simulink library "ddm"  (R2021b)
settings: Solver=VariableStepAuto  StartTime=0.0  StopTime=10.0  RelTol=1e-3
undefined symbols (not defined in the file or in its folder): ENUM_ADASACCSTA_ERROR, ENUM_ADASACCSTA_OFF, ENUM_ADASACCSTA_STANDBY, ENUM_ADASISASTA_OFF, ENUM_ALLOWMOV_ALLOWREADY, ENUM_APS, ENUM_BRKSTA_ERROR, ENUM_BRKSTA_OFF, ENUM_BRKSTA_ON, ENUM_CHGPREACTERRSTA_OBCPRE, ENUM_DCDCFAULTSTA_ANYFAULTLV1, ENUM_DCDCFAULTSTA_ANYFAULTLV2, ENUM_DRIVETRAIN_AWD, ENUM_DRIVETRAIN_FWD, ENUM_DRIVETRAIN_RWD, ENUM_DRSEATSTA_INVALID, ENUM_EDUDRTSTA_NORMAL, ENUM_EPBSTA_APPLIED, ENUM_EPBSTA_RELEASED, ENUM_HVBATTREADYPRE_READY, ENUM_MCUWARN_LV0, ENUM_MCUWARN_LV1, ENUM_MCUWARN_LV2, ENUM_MCUWARN_LV3, ENUM_MCUWARN_NOERROR, ENUM_OBCFAULTSTA_ANYFAULT, ENUM_PAS_R2F2, ENUM_PDFAULT_BATTPDFAIL, ENUM_PDFAULT_DCDCDISABLE, ENUM_PDFAULT_MCUDISABLE, ENUM_PDFAULT_MCUDISCHRG, ENUM_POWERSTA_OFF, ENUM_POWERSTA_ON, ENUM_POWERSTA_READY, ENUM_POWERSTA_STANDBY, ENUM_PRESSINDI_LOW, ENUM_PUFAULT_BATTUPFAIL, ENUM_PUFAULT_DCDCENABLEFAIL, ENUM_PUFAULT_PRECHRGCHKFAIL, ENUM_PUFAULT_SAFETYCHKFAIL, ENUM_PUSTATE_COMPLETED, ENUM_PWRSTASW_OFF, ENUM_PWRSTASW_OFFA, ENUM_PWRSTASW_OFFCHVCHRG, ENUM_PWRSTASW_OFFCLVCHRG, ENUM_PWRSTASW_ON, ENUM_PWRSTASW_ONHVCHRG, ENUM_PWRSTASW_READY, ENUM_PWRSTASW_STANDBY, ENUM_RANGESTA_12IN, ENUM_RANGESTA_12OUT, ENUM_SHIFTCOMMAND_D, ENUM_SHIFTCOMMAND_N, ENUM_SHIFTCOMMAND_P, ENUM_SHIFTCOMMAND_R, ENUM_ZONEMALFUNLV_1ST, ENUM_ZONEMALFUNLV_2ND, ENUM_ZONEMALFUNLV_3RD, ENUM_ZONEMALFUNLV_4TH, ENUM_ZONESPDCTRLMODE_ACC ... (+832)
libraries: hcu_lib x738, $bdroot x26, simulink x7
(part 13 of 25)

== system ddm/DDM/DDM/PMM/Comm err/FDC lost communication with EPAS2 ==
  note: Fail Safe After Decision
  note: Test Pass Criteria
  note: Diagnostics and Fault Handling
  note: Test Detection Criteria
  note: Fail Safe During Detection
  note: Release Condition After Failure Decision
  note: Release Condition During Failure Detection
  task_time_s : Inport
  VPMM_PowerSta_enum : Inport  Port=2
  VPMM_PwrStaSW_enum : Inport  Port=3
  VDDM_C1EPAS2LCChk_flg : Inport  Port=4
  No_CAN1_BUS_OFF : Inport  Port=5
  DTC_clear_request : Inport  Port=6
  Constant15 : Constant  Value=KDDM_C1EPAS2LCCFSSW_flg
  Constant16 : Constant  Value=TRUE
  Constant18 : Constant  Value=KDDM_C1EPAS2LCPassTO_s
  Constant19 : Constant  Value=KDDM_C1EPAS2LCPassTO_s
  Constant{2,21,25,27} (4 alike) : Constant  Value=FALSE
  Constant20 : Constant  Value=KDDM_C1EPAS2LCDFSSW_flg
  Constant24 : Constant  Value=TRUE
  Constant26 : Constant  Value=ENUM_PWRSTASW_OFF
  Constant28 : Constant  Value=ENUM_PWRSTASW_OFF
  Constant3 : Constant  Value=TRUE
  Constant4 : Constant  Value=ENUM_POWERSTA_OFF
  Constant40 : Constant  Value=KDDM_C1EPAS2LCDTC_cnt
  Constant41 : Constant  Value=KDDM_C1EPAS2LCDetTO_s
  Constant46 : Constant  Value=KDDM_C1EPAS2LCDetSW_flg
  Constant48 : Constant  Value=KDDM_C1EPAS2LCDTC_cnt
  Constant5 : Constant  Value=KDDM_C1EPAS2LCPassSW_flg
  DTC_Couter : hcu_lib/Basic_Blocks/DTC_Couter
  DTC_Info : hcu_lib/Basic_Blocks/DTC_Info
  Data Type Conversion1 : DataTypeConversion  OutDataTypeStr=uint8
  Equal : RelationalOperator  Operator=~=  OutDataTypeStr=boolean  RndMeth=Simplest
  Equal2 : RelationalOperator  Operator=~=  OutDataTypeStr=boolean  RndMeth=Simplest
  Equal3 : RelationalOperator  OutDataTypeStr=boolean  RndMeth=Simplest
  Equal4 : RelationalOperator  Operator===  OutDataTypeStr=boolean  RndMeth=Simplest
  Goto19 : Goto  Commented=on  GotoTag=EDriveSysErr_VCUErr_flg
  Logical Operator{2,5,12,15,18..19} (6 alike) : Logic  AllPortsSameDT=off  OutDataTypeStr=boolean
  Logical Operator3 : Logic  Operator=OR  AllPortsSameDT=off  OutDataTypeStr=boolean
  Logical Operator6 : Logic  Operator=NOT  AllPortsSameDT=off  OutDataTypeStr=boolean
  Logical Operator8 : Logic  Operator=OR  AllPortsSameDT=off  OutDataTypeStr=boolean
  Relay : Relay  OnSwitchValue=ONE_INT  OffSwitchValue=ZERO_INT
  SR_Latch1 : Subsystem  mask(SR_Latch){}
      mask help: SR latch function.
  SR_Latch3 : hcu_lib/Basic_Blocks/SR_Latch
  SR_Latch4 : hcu_lib/Basic_Blocks/SR_Latch
  Switch{,1,4..6} (5 alike) : Switch  Criteria=u2 ~= 0
  Test Detection Criteria : hcu_lib/Basic_Blocks/Test Detection Criteria
  Timer1 : hcu_lib/Basic_Blocks/Timer
  VDDM_C1EPAS2LCDTC_raw32 : Outport
  VDDM_C1EPAS2LCCFS_flg : Outport  Port=2
  wires:
  Constant2/1 -> Switch1/1
  Switch5/1 -> Switch1/3, [VDDM_xxx_flg]
  Switch1/1 -> Test Detection Criteria/1
  [DTC_clear_request] -> Switch1/2
  [DTC_clear_request] -> DTC_Info/4
  Constant41/1 -> Test Detection Criteria/4
  [VDDM_C1EPAS2LCPass_flg] -> DTC_Info/2
  [VDDM_C1EPAS2LCDet_flg] -> DTC_Info/1
  [VDDM_C1EPAS2LCCFS_flg] -> SR_Latch3/2
  [VDDM_C1EPAS2LCCFS_flg] -> VDDM_C1EPAS2LCCFS_flg/1, DTC_Info/3
  DTC_Info/1 -> VDDM_C1EPAS2LCDTC_raw32/1  "VDDM_C1EPAS2LCDTC_raw32"
  [task_time_s] -> Timer1/3
  [VPMM_PwrStaSW_enum] -> Equal2/1
  [VPMM_PwrStaSW_enum] -> Equal/1
  [VPMM_PowerSta_enum] -> Equal4/1
  Constant4/1 -> Equal4/2
  [VDDM_C1EPAS2LCPass_flg] -> Logical Operator3/1
  Constant18/1 -> Timer1/4
  [VDDM_C1EPAS2LCDet_flg] -> Logical Operator19/1
  Equal3/1 -> SR_Latch1/1(set)
  Logical Operator18/1 -> [VDDM_C1EPAS2LCCFS_flg]
  Switch6/1 -> Timer1/2, Logical Operator6/1
  SR_Latch1/1(latched) -> [VDDM_C1EPAS2LCPass_flg]
  Constant48/1 -> DTC_Couter/3
  SR_Latch4/1 -> Logical Operator18/1
  Constant28/1 -> Equal2/2
  DTC_Couter/2 -> Data Type Conversion1/1
  [VDDM_C1EPAS2LCChk_flg] -> Switch5/1
  Logical Operator15/1 -> DTC_Couter/2
  Logical Operator3/1 -> Logical Operator15/1
  Logical Operator8/1 -> Switch4/2
  Constant15/1 -> Logical Operator18/2
  [VDDM_C1EPAS2LCChk_flg] -> Switch6/1
  Switch4/1 -> [VDDM_C1EPAS2LCCFSRls_flg]
  Logical Operator19/1 -> DTC_Couter/1
  Constant25/1 -> Switch4/3
  Equal2/1 -> Logical Operator5/2
  Constant20/1 -> Logical Operator12/1
  [VDDM_C1EPAS2LCCFS_flg] -> Switch/2
  Constant21/1 -> Switch/3
  DTC_Couter/1 -> SR_Latch4/1
  Logical Operator12/1 -> [VDDM_C1EPAS2LCDFS_flg]
  Constant40/1 -> Test Detection Criteria/3
  [VDDM_xxx_flg] -> SR_Latch1/2(reset)
  [No_CAN1_BUS_OFF] -> Logical Operator5/1
  [VDDM_C1EPAS2LCCFSRls_flg] -> Logical Operator3/2
  Relay/1 -> SR_Latch3/1
  Switch/1 -> Goto19/1
  Logical Operator5/1 -> Switch6/2
  Logical Operator2/1 -> Switch5/2
  Constant24/1 -> Switch4/1
  Constant46/1 -> Logical Operator19/2
  SR_Latch3/1 -> Logical Operator12/2
  Constant5/1 -> Logical Operator15/2
  [VDDM_C1EPAS2LCCFSRls_flg] -> SR_Latch4/2
  Constant26/1 -> Equal/2
  [DTC_clear_request] -> Logical Operator8/2
  Data Type Conversion1/1 -> [VDDM_C1EPAS2LCDTC_cnt]  "VDDM_C1EPAS2LCDTC_cnt"
  [No_CAN1_BUS_OFF] -> Logical Operator2/1
  Constant27/1 -> Switch5/3
  Timer1/1 -> Equal3/1
  Equal4/1 -> Logical Operator8/1
  Equal/1 -> Logical Operator2/2
  [task_time_s] -> Test Detection Criteria/2
  Logical Operator6/1 -> Timer1/1
  [VDDM_C1EPAS2LCDTC_cnt] -> Relay/1
  Constant16/1 -> Switch6/3
  Constant19/1 -> Equal3/2
  Constant3/1 -> Switch/1
  No_CAN1_BUS_OFF/1 -> [No_CAN1_BUS_OFF]
  DTC_clear_request/1 -> [DTC_clear_request]
  task_time_s/1 -> [task_time_s]
  VDDM_C1EPAS2LCChk_flg/1 -> [VDDM_C1EPAS2LCChk_flg]
  VPMM_PwrStaSW_enum/1 -> [VPMM_PwrStaSW_enum]
  VPMM_PowerSta_enum/1 -> [VPMM_PowerSta_enum]
  Test Detection Criteria/1 -> [VDDM_C1EPAS2LCDet_flg]  "VDDM_C1EPAS2LCDet_flg"

== system ddm/DDM/DDM/PMM/Comm err/The CAN signal between VCU and ABM1 is discontinuous ==
  note: Fail Safe During Detection
  note: Diagnostics and Fault Handling
  note: Test Pass Criteria
  note: Test Detection Criteria
  note: Release Condition During Failure Detection
  note: Fail Safe After Decision
  note: Release Condition After Failure Decision
  task_time_s : Inport
  VPMM_PowerSta_enum : Inport  Port=2
  VPMM_PwrStaSW_enum : Inport  Port=3
  VDDM_C1ABM1RCChk_flg : Inport  Port=4
  VDDM_C1ABM1LCCFS_flg : Inport  Port=5
  No_CAN1_BUS_OFF : Inport  Port=6
  DTC_clear_request : Inport  Port=7
  Constant15 : Constant  Value=KDDM_C1ABM1RCCFSSW_flg
  Constant16 : Constant  Value=TRUE
  Constant18 : Constant  Value=KDDM_C1ABM1RCPassTO_s
  Constant19 : Constant  Value=KDDM_C1ABM1RCPassTO_s
  Constant{2,21,25,27} (4 alike) : Constant  Value=FALSE
  Constant20 : Constant  Value=KDDM_C1ABM1RCDFSSW_flg
  Constant24 : Constant  Value=TRUE
  Constant26 : Constant  Value=ENUM_PWRSTASW_OFF
  Constant28 : Constant  Value=ENUM_PWRSTASW_OFF
  Constant3 : Constant  Value=TRUE
  Constant4 : Constant  Value=ENUM_POWERSTA_OFF
  Constant40 : Constant  Value=KDDM_C1ABM1RCDTC_cnt
  Constant41 : Constant  Value=KDDM_C1ABM1RCDetTO_s
  Constant46 : Constant  Value=KDDM_C1ABM1RCDetSW_flg
  Constant48 : Constant  Value=KDDM_C1ABM1RCDTC_cnt
  Constant5 : Constant  Value=KDDM_C1ABM1RCPassSW_flg
  DTC_Couter : hcu_lib/Basic_Blocks/DTC_Couter
  DTC_Info : hcu_lib/Basic_Blocks/DTC_Info
  Data Type Conversion1 : DataTypeConversion  OutDataTypeStr=uint8
  Equal : RelationalOperator  Operator=~=  OutDataTypeStr=boolean  RndMeth=Simplest
  Equal2 : RelationalOperator  Operator=~=  OutDataTypeStr=boolean  RndMeth=Simplest
  Equal3 : RelationalOperator  OutDataTypeStr=boolean  RndMeth=Simplest
  Equal4 : RelationalOperator  Operator===  OutDataTypeStr=boolean  RndMeth=Simplest
  Logical Operator1 : Logic  Operator=NOT  AllPortsSameDT=off  OutDataTypeStr=boolean
  Logical Operator{12,15,18..19} (4 alike) : Logic  AllPortsSameDT=off  OutDataTypeStr=boolean
  Logical Operator2 : Logic  Inputs=3  AllPortsSameDT=off  OutDataTypeStr=boolean
  Logical Operator3 : Logic  Operator=OR  AllPortsSameDT=off  OutDataTypeStr=boolean
  Logical Operator4 : Logic  Operator=NOT  AllPortsSameDT=off  OutDataTypeStr=boolean
  Logical Operator5 : Logic  Inputs=3  AllPortsSameDT=off  OutDataTypeStr=boolean
  Logical Operator6 : Logic  Operator=NOT  AllPortsSameDT=off  OutDataTypeStr=boolean
  Logical Operator8 : Logic  Operator=OR  AllPortsSameDT=off  OutDataTypeStr=boolean
  Relay : Relay  OnSwitchValue=ONE_INT  OffSwitchValue=ZERO_INT
  SR_Latch1 : Subsystem  mask(SR_Latch){}
      mask help: SR latch function.
  SR_Latch3 : hcu_lib/Basic_Blocks/SR_Latch
  SR_Latch4 : hcu_lib/Basic_Blocks/SR_Latch
  Switch{,1,4..6} (5 alike) : Switch  Criteria=u2 ~= 0
  Test Detection Criteria : hcu_lib/Basic_Blocks/Test Detection Criteria
  Timer1 : hcu_lib/Basic_Blocks/Timer
  VDDM_C1ABM1RCDTC_raw32 : Outport
  RC_EDriveSysErr_VCUErr_flg : Outport  Port=2
  wires:
  task_time_s/1 -> [task_time_s]
  VDDM_C1ABM1RCChk_flg/1 -> [VDDM_C1ABM1RCChk_flg]
  VPMM_PwrStaSW_enum/1 -> [VPMM_PwrStaSW_enum]
  VPMM_PowerSta_enum/1 -> [VPMM_PowerSta_enum]
  VDDM_C1ABM1LCCFS_flg/1 -> [VDDM_C1ABM1LCCFS_flg]
  No_CAN1_BUS_OFF/1 -> [No_CAN1_BUS_OFF]
  DTC_clear_request/1 -> [DTC_clear_request]
  Equal2/1 -> Logical Operator5/2
  SR_Latch1/1(latched) -> [VDDM_C1ABM1RCPass_flg]
  SR_Latch4/1 -> Logical Operator18/1
  Constant20/1 -> Logical Operator12/1
  Logical Operator19/1 -> DTC_Couter/1
  Constant48/1 -> DTC_Couter/3
  [No_CAN1_BUS_OFF] -> Logical Operator5/1
  Data Type Conversion1/1 -> [VDDM_C1ABM1RCDTC_cnt]  "VDDM_C1ABM1RCDTC_cnt"
  Constant27/1 -> Switch5/3
  Switch6/1 -> Logical Operator6/1, Timer1/2
  Switch4/1 -> [VDDM_C1ABM1RCCFSRls_flg]
  Constant24/1 -> Switch4/1
  [VDDM_C1ABM1RCCFS_flg] -> Switch/2
  Constant5/1 -> Logical Operator15/2
  Constant3/1 -> Switch/1
  Constant18/1 -> Timer1/4
  [VDDM_C1ABM1LCCFS_flg] -> Logical Operator1/1
  Test Detection Criteria/1 -> [VDDM_C1ABM1RCDet_flg]  "VDDM_C1ABM1RCDet_flg"
  Constant46/1 -> Logical Operator19/2
  SR_Latch3/1 -> Logical Operator12/2
  Logical Operator4/1 -> Logical Operator5/3
  [VDDM_C1ABM1RCChk_flg] -> Switch5/1
  Constant40/1 -> Test Detection Criteria/3
  Constant26/1 -> Equal/2
  Logical Operator3/1 -> Logical Operator15/1
  [VDDM_C1ABM1RCDTC_cnt] -> Relay/1
  Constant19/1 -> Equal3/2
  Equal4/1 -> Logical Operator8/1
  [No_CAN1_BUS_OFF] -> Logical Operator2/1
  Constant25/1 -> Switch4/3
  Logical Operator2/1 -> Switch5/2
  Constant16/1 -> Switch6/3
  Logical Operator12/1 -> [VDDM_C1ABM1RCDFS_flg]
  [DTC_clear_request] -> Logical Operator8/2
  Relay/1 -> SR_Latch3/1
  Constant21/1 -> Switch/3
  Switch/1 -> [EDriveSysErr_VCUErr_flg]
  [VDDM_C1ABM1RCCFSRls_flg] -> Logical Operator3/2
  [VDDM_xxx_flg] -> SR_Latch1/2(reset)
  [VDDM_C1ABM1LCCFS_flg] -> Logical Operator4/1
  [task_time_s] -> Test Detection Criteria/2
  Logical Operator1/1 -> Logical Operator2/3
  Equal3/1 -> SR_Latch1/1(set)
  Timer1/1 -> Equal3/1
  [VDDM_C1ABM1RCChk_flg] -> Switch6/1
  Constant15/1 -> Logical Operator18/2
  Logical Operator6/1 -> Timer1/1
  Logical Operator5/1 -> Switch6/2
  Constant28/1 -> Equal2/2
  DTC_Couter/1 -> SR_Latch4/1
  Equal/1 -> Logical Operator2/2
  Logical Operator15/1 -> DTC_Couter/2
  [VDDM_C1ABM1RCDet_flg] -> Logical Operator19/1
  Logical Operator18/1 -> [VDDM_C1ABM1RCCFS_flg]
  Logical Operator8/1 -> Switch4/2
  Constant4/1 -> Equal4/2
  [VDDM_C1ABM1RCCFSRls_flg] -> SR_Latch4/2
  DTC_Couter/2 -> Data Type Conversion1/1
  [VDDM_C1ABM1RCPass_flg] -> Logical Operator3/1
  [EDriveSysErr_VCUErr_flg] -> RC_EDriveSysErr_VCUErr_flg/1
  [VPMM_PowerSta_enum] -> Equal4/1
  [VPMM_PwrStaSW_enum] -> Equal/1
  [VPMM_PwrStaSW_enum] -> Equal2/1
  [task_time_s] -> Timer1/3
  DTC_Info/1 -> VDDM_C1ABM1RCDTC_raw32/1  "VDDM_C1ABM1RCDTC_raw32"
  [VDDM_C1ABM1RCPass_flg] -> DTC_Info/2
  [VDDM_C1ABM1RCCFS_flg] -> DTC_Info/3
  [VDDM_C1ABM1RCCFS_flg] -> SR_Latch3/2
  [VDDM_C1ABM1RCDet_flg] -> DTC_Info/1
  Constant41/1 -> Test Detection Criteria/4
  [DTC_clear_request] -> DTC_Info/4
  [DTC_clear_request] -> Switch1/2
  Switch1/1 -> Test Detection Criteria/1
  Switch5/1 -> [VDDM_xxx_flg], Switch1/3
  Constant2/1 -> Switch1/1

== system ddm/DDM/DDM/PMM/Comm err/The CAN signal between VCU and ABM1 is incomplete ==
  note: Diagnostics and Fault Handling
  note: Fail Safe During Detection
  note: Release Condition After Failure Decision
  note: Fail Safe After Decision
  note: Release Condition During Failure Detection
  note: Test Detection Criteria
  note: Test Pass Criteria
  task_time_s : Inport
  VPMM_PowerSta_enum : Inport  Port=2
  VPMM_PwrStaSW_enum : Inport  Port=3
  VDDM_C1ABM1CSChk_flg : Inport  Port=4
  VDDM_C1ABM1LCCFS_flg : Inport  Port=5
  No_CAN1_BUS_OFF : Inport  Port=6
  DTC_clear_request : Inport  Port=7
  Constant15 : Constant  Value=KDDM_C1ABM1CSCFSSW_flg
  Constant16 : Constant  Value=TRUE
  Constant18 : Constant  Value=KDDM_C1ABM1CSPassTO_s
  Constant19 : Constant  Value=KDDM_C1ABM1CSPassTO_s
  Constant{2,21,25,27} (4 alike) : Constant  Value=FALSE
  Constant20 : Constant  Value=KDDM_C1ABM1CSDFSSW_flg
  Constant24 : Constant  Value=TRUE
  Constant26 : Constant  Value=ENUM_PWRSTASW_OFF
  Constant28 : Constant  Value=ENUM_PWRSTASW_OFF
  Constant3 : Constant  Value=TRUE
  Constant4 : Constant  Value=ENUM_POWERSTA_OFF
  Constant40 : Constant  Value=KDDM_C1ABM1CSDTC_cnt
  Constant41 : Constant  Value=KDDM_C1ABM1CSDetTO_s
  Constant46 : Constant  Value=KDDM_C1ABM1CSDetSW_flg
  Constant48 : Constant  Value=KDDM_C1ABM1CSDTC_cnt
  Constant5 : Constant  Value=KDDM_C1ABM1CSPassSW_flg
  DTC_Couter : hcu_lib/Basic_Blocks/DTC_Couter
  DTC_Info : hcu_lib/Basic_Blocks/DTC_Info
  Data Type Conversion1 : DataTypeConversion  OutDataTypeStr=uint8
  Equal : RelationalOperator  Operator=~=  OutDataTypeStr=boolean  RndMeth=Simplest
  Equal2 : RelationalOperator  Operator=~=  OutDataTypeStr=boolean  RndMeth=Simplest
  Equal3 : RelationalOperator  OutDataTypeStr=boolean  RndMeth=Simplest
  Equal4 : RelationalOperator  Operator===  OutDataTypeStr=boolean  RndMeth=Simplest
  Logical Operator1 : Logic  Operator=NOT  AllPortsSameDT=off  OutDataTypeStr=boolean
  Logical Operator{12,15,18..19} (4 alike) : Logic  AllPortsSameDT=off  OutDataTypeStr=boolean
  Logical Operator2 : Logic  Inputs=3  AllPortsSameDT=off  OutDataTypeStr=boolean
  Logical Operator3 : Logic  Operator=OR  AllPortsSameDT=off  OutDataTypeStr=boolean
  Logical Operator4 : Logic  Operator=NOT  AllPortsSameDT=off  OutDataTypeStr=boolean
  Logical Operator5 : Logic  Inputs=3  AllPortsSameDT=off  OutDataTypeStr=boolean
  Logical Operator6 : Logic  Operator=NOT  AllPortsSameDT=off  OutDataTypeStr=boolean
  Logical Operator8 : Logic  Operator=OR  AllPortsSameDT=off  OutDataTypeStr=boolean
  Relay : Relay  OnSwitchValue=ONE_INT  OffSwitchValue=ZERO_INT
  SR_Latch1 : Subsystem  mask(SR_Latch){}
      mask help: SR latch function.
  SR_Latch3 : hcu_lib/Basic_Blocks/SR_Latch
  SR_Latch4 : hcu_lib/Basic_Blocks/SR_Latch
  Switch{,1,4..6} (5 alike) : Switch  Criteria=u2 ~= 0
  Test Detection Criteria : hcu_lib/Basic_Blocks/Test Detection Criteria
  Timer1 : hcu_lib/Basic_Blocks/Timer
  VDDM_C1ABM1CSDTC_raw32 : Outport
  CS_EDriveSysErr_VCUErr_flg : Outport  Port=2
  wires:
  VDDM_C1ABM1LCCFS_flg/1 -> [VDDM_C1ABM1LCCFS_flg]
  VPMM_PowerSta_enum/1 -> [VPMM_PowerSta_enum]
  VPMM_PwrStaSW_enum/1 -> [VPMM_PwrStaSW_enum]
  VDDM_C1ABM1CSChk_flg/1 -> [VDDM_C1ABM1CSChk_flg]
  task_time_s/1 -> [task_time_s]
  DTC_clear_request/1 -> [DTC_clear_request]
  No_CAN1_BUS_OFF/1 -> [No_CAN1_BUS_OFF]
  SR_Latch4/1 -> Logical Operator18/1
  [VDDM_C1ABM1CSPass_flg] -> Logical Operator3/1
  DTC_Couter/2 -> Data Type Conversion1/1
  [VDDM_C1ABM1CSCFSRls_flg] -> SR_Latch4/2
  Constant4/1 -> Equal4/2
  [VDDM_C1ABM1CSDet_flg] -> Logical Operator19/1
  Logical Operator18/1 -> [VDDM_C1ABM1CSCFS_flg]
  Logical Operator15/1 -> DTC_Couter/2
  Equal2/1 -> Logical Operator5/2
  SR_Latch1/1(latched) -> [VDDM_C1ABM1CSPass_flg]
  Test Detection Criteria/1 -> [VDDM_C1ABM1CSDet_flg]  "VDDM_C1ABM1CSDet_flg"
  SR_Latch3/1 -> Logical Operator12/2
  [VDDM_C1ABM1LCCFS_flg] -> Logical Operator1/1
  Constant18/1 -> Timer1/4
  Logical Operator8/1 -> Switch4/2
  [VDDM_C1ABM1CSCFS_flg] -> Switch/2
  Constant5/1 -> Logical Operator15/2
  Constant24/1 -> Switch4/1
  Constant27/1 -> Switch5/3
  Switch4/1 -> [VDDM_C1ABM1CSCFSRls_flg]
  Switch6/1 -> Logical Operator6/1, Timer1/2
  Data Type Conversion1/1 -> [VDDM_C1ABM1CSDTC_cnt]  "VDDM_C1ABM1CSDTC_cnt"
  Constant20/1 -> Logical Operator12/1
  Logical Operator19/1 -> DTC_Couter/1
  DTC_Couter/1 -> SR_Latch4/1
  Constant28/1 -> Equal2/2
  Constant15/1 -> Logical Operator18/2
  [VDDM_C1ABM1CSChk_flg] -> Switch6/1
  Equal3/1 -> SR_Latch1/1(set)
  Constant48/1 -> DTC_Couter/3
  [task_time_s] -> Test Detection Criteria/2
  Logical Operator1/1 -> Logical Operator2/3
  Logical Operator5/1 -> Switch6/2
  [VDDM_C1ABM1LCCFS_flg] -> Logical Operator4/1
  [VDDM_xxx_flg] -> SR_Latch1/2(reset)
  [VDDM_C1ABM1CSCFSRls_flg] -> Logical Operator3/2
  Constant46/1 -> Logical Operator19/2
  Switch/1 -> [EDriveSysErr_VCUErr_flg]
  Constant21/1 -> Switch/3
  Logical Operator6/1 -> Timer1/1
  [DTC_clear_request] -> Logical Operator8/2
  Equal/1 -> Logical Operator2/2
  Logical Operator12/1 -> [VDDM_C1ABM1CSDFS_flg]
  Relay/1 -> SR_Latch3/1
  [No_CAN1_BUS_OFF] -> Logical Operator5/1
  Logical Operator2/1 -> Switch5/2
  Constant25/1 -> Switch4/3
  [No_CAN1_BUS_OFF] -> Logical Operator2/1
  Equal4/1 -> Logical Operator8/1
  Constant26/1 -> Equal/2
  Timer1/1 -> Equal3/1
  Logical Operator3/1 -> Logical Operator15/1
  Logical Operator4/1 -> Logical Operator5/3
  [VDDM_C1ABM1CSDTC_cnt] -> Relay/1
  [VDDM_C1ABM1CSChk_flg] -> Switch5/1
  Constant16/1 -> Switch6/3
  Constant40/1 -> Test Detection Criteria/3
  Constant19/1 -> Equal3/2
  Constant3/1 -> Switch/1
  [EDriveSysErr_VCUErr_flg] -> CS_EDriveSysErr_VCUErr_flg/1
  [VPMM_PowerSta_enum] -> Equal4/1
  [VPMM_PwrStaSW_enum] -> Equal/1
  [VPMM_PwrStaSW_enum] -> Equal2/1
  [task_time_s] -> Timer1/3
  DTC_Info/1 -> VDDM_C1ABM1CSDTC_raw32/1  "VDDM_C1ABM1CSDTC_raw32"
  [VDDM_C1ABM1CSCFS_flg] -> DTC_Info/3
  [VDDM_C1ABM1CSCFS_flg] -> SR_Latch3/2
  [VDDM_C1ABM1CSPass_flg] -> DTC_Info/2
  [VDDM_C1ABM1CSDet_flg] -> DTC_Info/1
  Constant41/1 -> Test Detection Criteria/4
  [DTC_clear_request] -> DTC_Info/4
  [DTC_clear_request] -> Switch1/2
  Switch1/1 -> Test Detection Criteria/1
  Switch5/1 -> [VDDM_xxx_flg], Switch1/3
  Constant2/1 -> Switch1/1

== system ddm/DDM/DDM/PMM/Comm err/The CAN signal between VCU and BMS1 is discontinuous ==
  note: Test Pass Criteria
  note: Release Condition After Failure Decision
  note: Diagnostics and Fault Handling
  note: Release Condition During Failure Detection
  note: Fail Safe After Decision
  note: Fail Safe During Detection
  note: Test Detection Criteria
  task_time_s : Inport
  VPMM_PowerSta_enum : Inport  Port=2
  VPMM_PwrStaSW_enum : Inport  Port=3
  VDDM_C3BMS1RCChk_flg : Inport  Port=4
  VDDM_C3BMS1LCCFS_flg : Inport  Port=5
  No_CAN3_BUS_OFF : Inport  Port=6
  DTC_clear_request : Inport  Port=7
  Constant15 : Constant  Value=KDDM_C3BMS1RCCFSSW_flg
  Constant{3,16,22,24} (4 alike) : Constant  Value=TRUE
  Constant18 : Constant  Value=KDDM_C3BMS1RCPassTO_s
  Constant19 : Constant  Value=KDDM_C3BMS1RCPassTO_s
  Constant{2,21,23,25,27} (5 alike) : Constant  Value=FALSE
  Constant20 : Constant  Value=KDDM_C3BMS1RCDFSSW_flg
  Constant26 : Constant  Value=ENUM_PWRSTASW_OFF
  Constant28 : Constant  Value=ENUM_PWRSTASW_OFF
  Constant4 : Constant  Value=ENUM_POWERSTA_OFF
  Constant40 : Constant  Value=KDDM_C3BMS1RCDTC_cnt
  Constant41 : Constant  Value=KDDM_C3BMS1RCDetTO_s
  Constant46 : Constant  Value=KDDM_C3BMS1RCDetSW_flg
  Constant48 : Constant  Value=KDDM_C3BMS1RCDTC_cnt
  Constant5 : Constant  Value=KDDM_C3BMS1RCPassSW_flg
  DTC_Couter : hcu_lib/Basic_Blocks/DTC_Couter
  DTC_Info : hcu_lib/Basic_Blocks/DTC_Info
  Data Type Conversion1 : DataTypeConversion  OutDataTypeStr=uint8
  Demux : Demux  Commented=on  Outputs=5
  Equal : RelationalOperator  Operator=~=  OutDataTypeStr=boolean  RndMeth=Simplest
  Equal2 : RelationalOperator  Operator=~=  OutDataTypeStr=boolean  RndMeth=Simplest
  Equal3 : RelationalOperator  OutDataTypeStr=boolean  RndMeth=Simplest
  Equal4 : RelationalOperator  Operator===  OutDataTypeStr=boolean  RndMeth=Simplest
  From19 : From  Commented=on  GotoTag=VDDM_C3BMS1RCDFS_flg
  Goto19 : Goto  Commented=on  GotoTag=VDDM_EDriveSysErrVCUErr_flg
  Logical Operator1 : Logic  Operator=NOT  AllPortsSameDT=off  OutDataTypeStr=boolean
  Logical Operator{12,15,18..19} (4 alike) : Logic  AllPortsSameDT=off  OutDataTypeStr=boolean
  Logical Operator2 : Logic  Inputs=3  AllPortsSameDT=off  OutDataTypeStr=boolean
  Logical Operator21 : Logic  Operator=OR  AllPortsSameDT=off  OutDataTypeStr=boolean
  Logical Operator3 : Logic  Operator=OR  AllPortsSameDT=off  OutDataTypeStr=boolean
  Logical Operator4 : Logic  Operator=NOT  AllPortsSameDT=off  OutDataTypeStr=boolean
  Logical Operator5 : Logic  Inputs=3  AllPortsSameDT=off  OutDataTypeStr=boolean
  Logical Operator6 : Logic  Operator=NOT  AllPortsSameDT=off  OutDataTypeStr=boolean
  Logical Operator8 : Logic  Operator=OR  AllPortsSameDT=off  OutDataTypeStr=boolean
  Relay : Relay  OnSwitchValue=ONE_INT  OffSwitchValue=ZERO_INT
  SR_Latch1 : Subsystem  mask(SR_Latch){}
      mask help: SR latch function.
  SR_Latch3 : hcu_lib/Basic_Blocks/SR_Latch
  SR_Latch4 : hcu_lib/Basic_Blocks/SR_Latch
  Switch{,1,4..7} (6 alike) : Switch  Criteria=u2 ~= 0
  Switch3 : Switch  Commented=on  Criteria=u2 ~= 0
  Test Detection Criteria1 : hcu_lib/Basic_Blocks/Test Detection Criteria
  Timer1 : hcu_lib/Basic_Blocks/Timer
  Unit Delay3 : UnitDelay  Commented=on  SampleTime=-1  HasFrameUpgradeWarning=on
  VDDM_C3BMS1RCDTC_raw32 : Outport
  wires:
  VPMM_PowerSta_enum/1 -> [VPMM_PowerSta_enum]
  VPMM_PwrStaSW_enum/1 -> [VPMM_PwrStaSW_enum]
  VDDM_C3BMS1RCChk_flg/1 -> [VDDM_C3BMS1RCChk_flg]
  task_time_s/1 -> [task_time_s]
  VDDM_C3BMS1LCCFS_flg/1 -> [VDDM_C3BMS1LCCFS_flg]
  No_CAN3_BUS_OFF/1 -> [No_CAN3_BUS_OFF]
  DTC_clear_request/1 -> [DTC_clear_request]
  [VDDM_C3BMS1LCCFS_flg] -> Logical Operator4/1
  [VDDM_C3BMS1LCCFS_flg] -> Logical Operator1/1
  Logical Operator5/1 -> Switch6/2
  [No_CAN3_BUS_OFF] -> Logical Operator5/1
  Demux/1 -> Unit Delay3/1
  Logical Operator1/1 -> Logical Operator2/3
  Constant46/1 -> Logical Operator19/2
  Constant20/1 -> Logical Operator12/1
  Constant15/1 -> Logical Operator18/2
  Logical Operator4/1 -> Logical Operator5/3
  Constant5/1 -> Logical Operator15/2
  Logical Operator15/1 -> DTC_Couter/2
  Logical Operator18/1 -> [VDDM_C3BMS1RCCFS_flg]
  SR_Latch4/1 -> Logical Operator18/1
  [VDDM_C3BMS1RCPass_flg] -> Logical Operator3/1
  Switch3/1 -> Demux/1
  DTC_Couter/1 -> SR_Latch4/1
  Data Type Conversion1/1 -> [VDDM_C3BMS1RCDTC_cnt]  "VDDM_C3BMS1RCDTC_cnt"
  Equal3/1 -> SR_Latch1/1(set)
  SR_Latch3/1 -> Logical Operator12/2
  Logical Operator3/1 -> Logical Operator15/1
  [VDDM_C3BMS1RCDFSRls_flg] -> Logical Operator21/1
  Constant18/1 -> Timer1/4
  Constant22/1 -> Switch7/1
  Constant4/1 -> Equal4/2
  Timer1/1 -> Equal3/1
  [VDDM_C3BMS1RCDet_flg] -> Logical Operator19/1
  [VDDM_C3BMS1RCCFSRls_flg] -> SR_Latch4/2
  Switch/1 -> Goto19/1
  Relay/1 -> SR_Latch3/1
  Logical Operator6/1 -> Timer1/1
  Constant24/1 -> Switch4/1
  [VDDM_C3BMS1RCPass_flg] -> Switch7/2
  DTC_Couter/2 -> Data Type Conversion1/1
  Constant48/1 -> DTC_Couter/3
  Equal4/1 -> Logical Operator8/1
  Logical Operator19/1 -> DTC_Couter/1
  Switch4/1 -> [VDDM_C3BMS1RCCFSRls_flg]
  SR_Latch1/1(latched) -> [VDDM_C3BMS1RCPass_flg]
  Constant28/1 -> Equal2/2
  Logical Operator12/1 -> [VDDM_C3BMS1RCDFS_flg]
  [No_CAN3_BUS_OFF] -> Logical Operator2/1
  Constant16/1 -> Switch6/3
  Constant27/1 -> Switch5/3
  [VDDM_C3BMS1RCDTC_cnt] -> Relay/1
  Logical Operator21/1 -> SR_Latch3/2
  Logical Operator8/1 -> Switch4/2
  From19/1 -> Switch3/2
  [DTC_clear_request] -> Logical Operator8/2
  Constant23/1 -> Switch7/3
  [VDDM_C3BMS1RCCFS_flg] -> Logical Operator21/2
  Constant21/1 -> Switch/3
  Constant25/1 -> Switch4/3
  [VDDM_C3BMS1RCChk_flg] -> Switch6/1
  [VDDM_xxx_flg] -> SR_Latch1/2(reset)
  Switch7/1 -> [VDDM_C3BMS1RCDFSRls_flg]
  Equal/1 -> Logical Operator2/2
  Logical Operator2/1 -> Switch5/2
  Constant19/1 -> Equal3/2
  Constant26/1 -> Equal/2
  [VDDM_C3BMS1RCChk_flg] -> Switch5/1
  [task_time_s] -> Test Detection Criteria1/2
  [VDDM_C3BMS1RCCFSRls_flg] -> Logical Operator3/2
  Constant40/1 -> Test Detection Criteria1/3
  Test Detection Criteria1/1 -> [VDDM_C3BMS1RCDet_flg]  "VDDM_C3BMS1RCDet_flg"
  Equal2/1 -> Logical Operator5/2
  Switch6/1 -> Logical Operator6/1, Timer1/2
  Constant3/1 -> Switch/1
  [VDDM_C3BMS1RCCFS_flg] -> Switch/2
  [VPMM_PowerSta_enum] -> Equal4/1
  [VPMM_PwrStaSW_enum] -> Equal/1
  [VPMM_PwrStaSW_enum] -> Equal2/1
  [task_time_s] -> Timer1/3
  [VDDM_C3BMS1RCPass_flg] -> DTC_Info/2
  [VDDM_C3BMS1RCCFS_flg] -> DTC_Info/3
  DTC_Info/1 -> VDDM_C3BMS1RCDTC_raw32/1  "VDDM_C3BMS1RCDTC_raw32"
  [VDDM_C3BMS1RCDet_flg] -> DTC_Info/1
  Constant41/1 -> Test Detection Criteria1/4
  [DTC_clear_request] -> DTC_Info/4
  [DTC_clear_request] -> Switch1/2
  Switch1/1 -> Test Detection Criteria1/1
  Switch5/1 -> [VDDM_xxx_flg], Switch1/3
  Constant2/1 -> Switch1/1

== system ddm/DDM/DDM/PMM/Comm err/The CAN signal between VCU and BMS1 is incomplete ==
  note: Release Condition After Failure Decision
  note: Fail Safe After Decision
  note: Test Detection Criteria
  note: Fail Safe During Detection
  note: Release Condition During Failure Detection
  note: Test Pass Criteria
  note: Diagnostics and Fault Handling
  task_time_s : Inport
  VPMM_PowerSta_enum : Inport  Port=2
  VPMM_PwrStaSW_enum : Inport  Port=3
  VDDM_C3BMS1CSChk_flg : Inport  Port=4
  VDDM_C3BMS1LCCFS_flg : Inport  Port=5
  No_CAN3_BUS_OFF : Inport  Port=6
  DTC_clear_request : Inport  Port=7
  Constant15 : Constant  Value=KDDM_C3BMS1CSCFSSW_flg
  Constant{3,16,22,24} (4 alike) : Constant  Value=TRUE
  Constant18 : Constant  Value=KDDM_C3BMS1CSPassTO_s
  Constant19 : Constant  Value=KDDM_C3BMS1CSPassTO_s
  Constant{2,21,23,25,27} (5 alike) : Constant  Value=FALSE
  Constant20 : Constant  Value=KDDM_C3BMS1CSDFSSW_flg
  Constant26 : Constant  Value=ENUM_PWRSTASW_OFF
  Constant28 : Constant  Value=ENUM_PWRSTASW_OFF
  Constant4 : Constant  Value=ENUM_POWERSTA_OFF
  Constant40 : Constant  Value=KDDM_C3BMS1CSDTC_cnt
  Constant41 : Constant  Value=KDDM_C3BMS1CSDetTO_s
  Constant46 : Constant  Value=KDDM_C3BMS1CSDetSW_flg
  Constant48 : Constant  Value=KDDM_C3BMS1CSDTC_cnt
  Constant5 : Constant  Value=KDDM_C3BMS1CSPassSW_flg
  DTC_Couter : hcu_lib/Basic_Blocks/DTC_Couter
  DTC_Info : hcu_lib/Basic_Blocks/DTC_Info
  Data Type Conversion1 : DataTypeConversion  OutDataTypeStr=uint8
  Demux : Demux  Commented=on  Outputs=5
  Equal : RelationalOperator  Operator=~=  OutDataTypeStr=boolean  RndMeth=Simplest
  Equal2 : RelationalOperator  Operator=~=  OutDataTypeStr=boolean  RndMeth=Simplest
  Equal3 : RelationalOperator  OutDataTypeStr=boolean  RndMeth=Simplest
  Equal4 : RelationalOperator  Operator===  OutDataTypeStr=boolean  RndMeth=Simplest
  From19 : From  Commented=on  GotoTag=VDDM_C3BMS1CSDFS_flg
  Goto19 : Goto  Commented=on  GotoTag=VDDM_EDriveSysErrVCUErr_flg
  Logical Operator1 : Logic  Operator=NOT  AllPortsSameDT=off  OutDataTypeStr=boolean
  Logical Operator{12,15,18..19} (4 alike) : Logic  AllPortsSameDT=off  OutDataTypeStr=boolean
  Logical Operator2 : Logic  Inputs=3  AllPortsSameDT=off  OutDataTypeStr=boolean
  Logical Operator21 : Logic  Operator=OR  AllPortsSameDT=off  OutDataTypeStr=boolean
  Logical Operator3 : Logic  Operator=OR  AllPortsSameDT=off  OutDataTypeStr=boolean
  Logical Operator4 : Logic  Operator=NOT  AllPortsSameDT=off  OutDataTypeStr=boolean
  Logical Operator5 : Logic  Inputs=3  AllPortsSameDT=off  OutDataTypeStr=boolean
  Logical Operator6 : Logic  Operator=NOT  AllPortsSameDT=off  OutDataTypeStr=boolean
  Logical Operator8 : Logic  Operator=OR  AllPortsSameDT=off  OutDataTypeStr=boolean
  Relay : Relay  OnSwitchValue=ONE_INT  OffSwitchValue=ZERO_INT
  SR_Latch1 : Subsystem  mask(SR_Latch){}
      mask help: SR latch function.
  SR_Latch3 : hcu_lib/Basic_Blocks/SR_Latch
  SR_Latch4 : hcu_lib/Basic_Blocks/SR_Latch
  Switch{,1,4..7} (6 alike) : Switch  Criteria=u2 ~= 0
  Switch3 : Switch  Commented=on  Criteria=u2 ~= 0
  Test Detection Criteria : hcu_lib/Basic_Blocks/Test Detection Criteria
  Timer1 : hcu_lib/Basic_Blocks/Timer
  Unit Delay3 : UnitDelay  Commented=on  SampleTime=-1  HasFrameUpgradeWarning=on
  VDDM_C3BMS1CSDTC_raw32 : Outport
  wires:
  task_time_s/1 -> [task_time_s]
  VDDM_C3BMS1CSChk_flg/1 -> [VDDM_C3BMS1CSChk_flg]
  VPMM_PwrStaSW_enum/1 -> [VPMM_PwrStaSW_enum]
  VPMM_PowerSta_enum/1 -> [VPMM_PowerSta_enum]
  VDDM_C3BMS1LCCFS_flg/1 -> [VDDM_C3BMS1LCCFS_flg]
  No_CAN3_BUS_OFF/1 -> [No_CAN3_BUS_OFF]
  DTC_clear_request/1 -> [DTC_clear_request]
  Constant26/1 -> Equal/2
  SR_Latch1/1(latched) -> [VDDM_C3BMS1CSPass_flg]
  [VDDM_xxx_flg] -> SR_Latch1/2(reset)
  Equal2/1 -> Logical Operator5/2
  Test Detection Criteria/1 -> [VDDM_C3BMS1CSDet_flg]  "VDDM_C3BMS1CSDet_flg"
  Logical Operator21/1 -> SR_Latch3/2
  [VDDM_C3BMS1CSChk_flg] -> Switch5/1
  Constant3/1 -> Switch/1
  Switch6/1 -> Logical Operator6/1, Timer1/2
  Equal4/1 -> Logical Operator8/1
  Constant20/1 -> Logical Operator12/1
  [VDDM_C3BMS1CSCFSRls_flg] -> Logical Operator3/2
  Logical Operator4/1 -> Logical Operator5/3
  [VDDM_C3BMS1CSChk_flg] -> Switch6/1
  Constant22/1 -> Switch7/1
  Constant40/1 -> Test Detection Criteria/3
  [DTC_clear_request] -> Logical Operator8/2
  Logical Operator15/1 -> DTC_Couter/2
  Logical Operator8/1 -> Switch4/2
  Constant4/1 -> Equal4/2
  Switch4/1 -> [VDDM_C3BMS1CSCFSRls_flg]
  Equal/1 -> Logical Operator2/2
  Constant23/1 -> Switch7/3
  Constant18/1 -> Timer1/4
  Switch7/1 -> [VDDM_C3BMS1CSDFSRls_flg]
  Constant25/1 -> Switch4/3
  Equal3/1 -> SR_Latch1/1(set)
  Logical Operator2/1 -> Switch5/2
  Logical Operator19/1 -> DTC_Couter/1
  Constant28/1 -> Equal2/2
  [No_CAN3_BUS_OFF] -> Logical Operator2/1
  SR_Latch3/1 -> Logical Operator12/2
  Logical Operator3/1 -> Logical Operator15/1
  [VDDM_C3BMS1CSDet_flg] -> Logical Operator19/1
  From19/1 -> Switch3/2
  Constant19/1 -> Equal3/2
  [VDDM_C3BMS1CSPass_flg] -> Logical Operator3/1
  [VDDM_C3BMS1CSPass_flg] -> Switch7/2
  Constant48/1 -> DTC_Couter/3
  [VDDM_C3BMS1CSCFS_flg] -> Logical Operator21/2
  [VDDM_C3BMS1CSDFSRls_flg] -> Logical Operator21/1
  Constant27/1 -> Switch5/3
  Logical Operator12/1 -> [VDDM_C3BMS1CSDFS_flg]
  Relay/1 -> SR_Latch3/1
  DTC_Couter/2 -> Data Type Conversion1/1
  Switch/1 -> Goto19/1
  [No_CAN3_BUS_OFF] -> Logical Operator5/1
  Data Type Conversion1/1 -> [VDDM_C3BMS1CSDTC_cnt]  "VDDM_C3BMS1CSDTC_cnt"
  [VDDM_C3BMS1CSCFS_flg] -> Switch/2
  [VDDM_C3BMS1CSCFSRls_flg] -> SR_Latch4/2
  DTC_Couter/1 -> SR_Latch4/1
  Constant15/1 -> Logical Operator18/2
  Constant16/1 -> Switch6/3
  Timer1/1 -> Equal3/1
  Logical Operator18/1 -> [VDDM_C3BMS1CSCFS_flg]
  [task_time_s] -> Test Detection Criteria/2
  Constant5/1 -> Logical Operator15/2
  Constant24/1 -> Switch4/1
  Logical Operator6/1 -> Timer1/1
  Switch3/1 -> Demux/1
  SR_Latch4/1 -> Logical Operator18/1
  [VDDM_C3BMS1LCCFS_flg] -> Logical Operator4/1
  Constant46/1 -> Logical Operator19/2
  [VDDM_C3BMS1CSDTC_cnt] -> Relay/1
  Logical Operator1/1 -> Logical Operator2/3
  Constant21/1 -> Switch/3
  [VDDM_C3BMS1LCCFS_flg] -> Logical Operator1/1
  Logical Operator5/1 -> Switch6/2
  Demux/1 -> Unit Delay3/1
  [VPMM_PowerSta_enum] -> Equal4/1
  [VPMM_PwrStaSW_enum] -> Equal/1
  [VPMM_PwrStaSW_enum] -> Equal2/1
  [task_time_s] -> Timer1/3
  DTC_Info/1 -> VDDM_C3BMS1CSDTC_raw32/1  "VDDM_C3BMS1CSDTC_raw32"
  [VDDM_C3BMS1CSCFS_flg] -> DTC_Info/3
  [VDDM_C3BMS1CSDet_flg] -> DTC_Info/1
  [VDDM_C3BMS1CSPass_flg] -> DTC_Info/2
  Constant41/1 -> Test Detection Criteria/4
  [DTC_clear_request] -> DTC_Info/4
  [DTC_clear_request] -> Switch1/2
  Switch1/1 -> Test Detection Criteria/1
  Switch5/1 -> [VDDM_xxx_flg], Switch1/3
  Constant2/1 -> Switch1/1

== system ddm/DDM/DDM/PMM/Comm err/The CAN signal between VCU and BMS6 is discontinuous ==
  note: Test Detection Criteria
  note: Test Pass Criteria
  note: Fail Safe After Decision
  note: Fail Safe During Detection
  note: Release Condition During Detection
  note: Release Condition After Decision
  note: Diagnostics and Fault Handling
  task_time_s : Inport
  VPMM_PowerSta_enum : Inport  Port=2
  VPMM_PwrStaSW_enum : Inport  Port=3
  VDDM_C3BMS6RCChk_flg : Inport  Port=4
  VDDM_C3BMS6LCCFS_flg : Inport  Port=5
  No_CAN3_BUS_OFF : Inport  Port=6
  DTC_clear_request : Inport  Port=7
  Constant{1,16,22,24} (4 alike) : Constant  Value=TRUE
  Constant10 : Constant  Value=ENUM_POWERSTA_OFF
  Constant11 : Constant  Value=KDDM_C3BMS6RCPassSW_flg
  Constant15 : Constant  Value=KDDM_C3BMS6RCCFSSW_flg
  Constant18 : Constant  Value=KDDM_C3BMS6RCPassTO_s
  Constant19 : Constant  Value=KDDM_C3BMS6RCPassTO_s
  Constant{2,4,21,23,25} (5 alike) : Constant  Value=FALSE
  Constant20 : Constant  Value=KDDM_C3BMS6RCDFSSW_flg
  Constant3 : Constant  Value=ENUM_PWRSTASW_OFF
  Constant40 : Constant  Value=KDDM_C3BMS6RCDTC_cnt
  Constant41 : Constant  Value=KDDM_C3BMS6RCDetTO_s
  Constant46 : Constant  Value=KDDM_C3BMS6RCDetSW_flg
  Constant48 : Constant  Value=KDDM_C3BMS6RCDTC_cnt
  Constant5 : Constant  Value=ENUM_PWRSTASW_OFF
  DTC_Couter : hcu_lib/Basic_Blocks/DTC_Couter
  DTC_Info : hcu_lib/Basic_Blocks/DTC_Info
  Data Type Conversion1 : DataTypeConversion  OutDataTypeStr=uint8
  Demux : Demux  Commented=on  Outputs=5
  Equal : RelationalOperator  Operator=~=  OutDataTypeStr=boolean  RndMeth=Simplest
  Equal2 : RelationalOperator  Operator=~=  OutDataTypeStr=boolean  RndMeth=Simplest
  Equal3 : RelationalOperator  OutDataTypeStr=boolean  RndMeth=Simplest
  Equal4 : RelationalOperator  Operator===  OutDataTypeStr=boolean  RndMeth=Simplest
  From12 : From  Commented=on  GotoTag=VDDM_C3BMS6RCDFS_flg
  Goto6 : Goto  Commented=on  GotoTag=VDDM_EDriveSysErrVCUErr_flg
  Logical Operator1 : Logic  Operator=NOT  AllPortsSameDT=off  OutDataTypeStr=boolean
  Logical Operator{12,15,18..19} (4 alike) : Logic  AllPortsSameDT=off  OutDataTypeStr=boolean
  Logical Operator2 : Logic  Inputs=3  AllPortsSameDT=off  OutDataTypeStr=boolean
  Logical Operator21 : Logic  Operator=OR  AllPortsSameDT=off  OutDataTypeStr=boolean
  Logical Operator3 : Logic  Operator=OR  AllPortsSameDT=off  OutDataTypeStr=boolean
  Logical Operator4 : Logic  Operator=NOT  AllPortsSameDT=off  OutDataTypeStr=boolean
  Logical Operator5 : Logic  Inputs=3  AllPortsSameDT=off  OutDataTypeStr=boolean
  Logical Operator6 : Logic  Operator=NOT  AllPortsSameDT=off  OutDataTypeStr=boolean
  Logical Operator8 : Logic  Operator=OR  AllPortsSameDT=off  OutDataTypeStr=boolean
  Relay : Relay  OnSwitchValue=ONE_INT  OffSwitchValue=ZERO_INT
  SR_Latch1 : Subsystem  mask(SR_Latch){}
      mask help: SR latch function.
  SR_Latch3 : hcu_lib/Basic_Blocks/SR_Latch
  SR_Latch4 : hcu_lib/Basic_Blocks/SR_Latch
  Switch{,2..6} (6 alike) : Switch  Criteria=u2 ~= 0
  Switch1 : Switch  Commented=on  Criteria=u2 ~= 0
  Test Detection Criteria : hcu_lib/Basic_Blocks/Test Detection Criteria
  Timer1 : hcu_lib/Basic_Blocks/Timer
  Unit Delay3 : UnitDelay  Commented=on  SampleTime=-1  HasFrameUpgradeWarning=on
  VDDM_C3BMS6RCDTC_raw32 : Outport
  VDDM_C3BMS6RCCFS_flg : Outport  Port=2
  wires:
  task_time_s/1 -> [task_time_s]
  VDDM_C3BMS6RCChk_flg/1 -> [VDDM_C3BMS6RCChk_flg]
  VPMM_PwrStaSW_enum/1 -> [VPMM_PwrStaSW_enum]
  VPMM_PowerSta_enum/1 -> [VPMM_PowerSta_enum]
  No_CAN3_BUS_OFF/1 -> [No_CAN3_BUS_OFF]
  Logical Operator2/1 -> Switch3/2
  [task_time_s] -> Test Detection Criteria/2
  Constant40/1 -> Test Detection Criteria/3
  Switch3/1 -> [VDDM_xxx_flg], Switch6/3
  Constant3/1 -> Equal/2
  Constant4/1 -> Switch3/3
  [VDDM_C3BMS6RCChk_flg] -> Switch3/1
  Equal/1 -> Logical Operator2/2
  [No_CAN3_BUS_OFF] -> Logical Operator2/1
  Constant5/1 -> Equal2/2
  SR_Latch1/1(latched) -> [VDDM_C3BMS6RCPass_flg]
  Equal3/1 -> SR_Latch1/1(set)
  Logical Operator6/1 -> Timer1/1
  Logical Operator5/1 -> Switch4/2
  Constant19/1 -> Equal3/2
  [VDDM_xxx_flg] -> SR_Latch1/2(reset)
  Switch4/1 -> Logical Operator6/1, Timer1/2
  [VDDM_C3BMS6RCChk_flg] -> Switch4/1
  Timer1/1 -> Equal3/1
  [No_CAN3_BUS_OFF] -> Logical Operator5/1
  Constant18/1 -> Timer1/4
  Equal2/1 -> Logical Operator5/2
  Constant16/1 -> Switch4/3
  [VDDM_C3BMS6RCCFS_flg] -> Switch/2
  Switch/1 -> Goto6/1
  Constant1/1 -> Switch/1
  Constant21/1 -> Switch/3
  [VDDM_C3BMS6RCPass_flg] -> Switch5/2
  Constant22/1 -> Switch5/1
  Switch5/1 -> [VDDM_C3BMS6RCDFSRls_flg]
  Constant23/1 -> Switch5/3
  Logical Operator8/1 -> Switch2/2
  Constant25/1 -> Switch2/3
  Switch2/1 -> [VDDM_C3BMS6RCCFSRls_flg]
  [DTC_clear_request] -> Logical Operator8/2
  Constant24/1 -> Switch2/1
  Constant10/1 -> Equal4/2
  Equal4/1 -> Logical Operator8/1
  From12/1 -> Switch1/2
  [VDDM_C3BMS6RCDTC_cnt] -> Relay/1
  Logical Operator21/1 -> SR_Latch3/2
  Logical Operator3/1 -> Logical Operator15/1
  [VDDM_C3BMS6RCDet_flg] -> Logical Operator19/1
  Relay/1 -> SR_Latch3/1
  DTC_Couter/2 -> Data Type Conversion1/1
  Constant48/1 -> DTC_Couter/3
  Logical Operator15/1 -> DTC_Couter/2
  Constant11/1 -> Logical Operator15/2
  Logical Operator19/1 -> DTC_Couter/1
  Constant46/1 -> Logical Operator19/2
  Data Type Conversion1/1 -> [VDDM_C3BMS6RCDTC_cnt]  "VDDM_C3BMS6RCDTC_cnt"
  DTC_Couter/1 -> SR_Latch4/1
  [VDDM_C3BMS6RCPass_flg] -> Logical Operator3/1
  [VDDM_C3BMS6RCCFS_flg] -> Logical Operator21/2
  [VDDM_C3BMS6RCCFSRls_flg] -> SR_Latch4/2
  SR_Latch4/1 -> Logical Operator18/1
  Logical Operator12/1 -> [VDDM_C3BMS6RCDFS_flg]
  Constant15/1 -> Logical Operator18/2
  [VDDM_C3BMS6RCDFSRls_flg] -> Logical Operator21/1
  SR_Latch3/1 -> Logical Operator12/2
  Constant20/1 -> Logical Operator12/1
  Logical Operator18/1 -> [VDDM_C3BMS6RCCFS_flg]
  Switch1/1 -> Demux/1
  [VDDM_C3BMS6RCCFSRls_flg] -> Logical Operator3/2
  Demux/1 -> Unit Delay3/1
  DTC_clear_request/1 -> [DTC_clear_request]
  VDDM_C3BMS6LCCFS_flg/1 -> [VDDM_C3BMS6LCCFS_flg]
  [VDDM_C3BMS6LCCFS_flg] -> Logical Operator1/1
  Logical Operator1/1 -> Logical Operator2/3
  [VDDM_C3BMS6LCCFS_flg] -> Logical Operator4/1
  Logical Operator4/1 -> Logical Operator5/3
  [VPMM_PwrStaSW_enum] -> Equal/1
  [VPMM_PowerSta_enum] -> Equal4/1
  [VPMM_PwrStaSW_enum] -> Equal2/1
  [task_time_s] -> Timer1/3
  [VDDM_C3BMS6RCCFS_flg] -> DTC_Info/3
  DTC_Info/1 -> VDDM_C3BMS6RCDTC_raw32/1  "VDDM_C3BMS6RCDTC_raw32"
  Test Detection Criteria/1 -> [VDDM_C3BMS6RCDet_flg]  "VDDM_C3BMS6RCDet_flg"
  Constant41/1 -> Test Detection Criteria/4
  [VDDM_C3BMS6RCDet_flg] -> DTC_Info/1
  [VDDM_C3BMS6RCPass_flg] -> DTC_Info/2
  [DTC_clear_request] -> DTC_Info/4
  Constant2/1 -> Switch6/1
  Switch6/1 -> Test Detection Criteria/1
  [DTC_clear_request] -> Switch6/2
  [VDDM_C3BMS6RCCFS_flg] -> VDDM_C3BMS6RCCFS_flg/1

== system ddm/DDM/DDM/PMM/Comm err/The CAN signal between VCU and BMS6 is incomplete ==
  note: Test Pass Criteria
  note: Release Condition After Decision
  note: Diagnostics and Fault Handling
  note: Release Condition During Detection
  note: Fail Safe After Decision
  note: Fail Safe During Detection
  note: Test Detection Criteria
  task_time_s : Inport
  VPMM_PowerSta_enum : Inport  Port=2
  VPMM_PwrStaSW_enum : Inport  Port=3
  VDDM_C3BMS6CSChk_flg : Inport  Port=4
  VDDM_C3BMS6LCCFS_flg : Inport  Port=5
  No_CAN3_BUS_OFF : Inport  Port=6
  DTC_clear_request : Inport  Port=7
  Constant1 : Constant  Value=ENUM_PWRSTASW_OFF
  Constant15 : Constant  Value=KDDM_C3BMS6CSCFSSW_flg
  Constant{3,16,22,24} (4 alike) : Constant  Value=TRUE
  Constant18 : Constant  Value=KDDM_C3BMS6CSPassTO_s
  Constant19 : Constant  Value=KDDM_C3BMS6CSPassTO_s
  Constant{2,21,23,25,28} (5 alike) : Constant  Value=FALSE
  Constant20 : Constant  Value=KDDM_C3BMS6CSDFSSW_flg
  Constant26 : Constant  Value=ENUM_PWRSTASW_OFF
  Constant4 : Constant  Value=ENUM_POWERSTA_OFF
  Constant40 : Constant  Value=KDDM_C3BMS6CSDTC_cnt
  Constant41 : Constant  Value=KDDM_C3BMS6CSDetTO_s
  Constant46 : Constant  Value=KDDM_C3BMS6CSDetSW_flg
  Constant48 : Constant  Value=KDDM_C3BMS6CSDTC_cnt
  Constant5 : Constant  Value=KDDM_C3BMS6CSPassSW_flg
  DTC_Couter : hcu_lib/Basic_Blocks/DTC_Couter
  DTC_Info : hcu_lib/Basic_Blocks/DTC_Info
  Data Type Conversion1 : DataTypeConversion  OutDataTypeStr=uint8
  Demux : Demux  Commented=on  Outputs=5
  Equal : RelationalOperator  Operator=~=  OutDataTypeStr=boolean  RndMeth=Simplest
  Equal1 : RelationalOperator  Operator=~=  OutDataTypeStr=boolean  RndMeth=Simplest
  Equal3 : RelationalOperator  OutDataTypeStr=boolean  RndMeth=Simplest
  Equal4 : RelationalOperator  Operator===  OutDataTypeStr=boolean  RndMeth=Simplest
  From13 : From  Commented=on  GotoTag=VDDM_C3BMS6CSDFS_flg
  Goto16 : Goto  Commented=on  GotoTag=VDDM_EDriveSysErrVCUErr_flg
  Logical Operator1 : Logic  Operator=NOT  AllPortsSameDT=off  OutDataTypeStr=boolean
  Logical Operator{12,15,18..19} (4 alike) : Logic  AllPortsSameDT=off  OutDataTypeStr=boolean
  Logical Operator2 : Logic  Inputs=3  AllPortsSameDT=off  OutDataTypeStr=boolean
  Logical Operator21 : Logic  Operator=OR  AllPortsSameDT=off  OutDataTypeStr=boolean
  Logical Operator3 : Logic  Operator=OR  AllPortsSameDT=off  OutDataTypeStr=boolean
  Logical Operator4 : Logic  Operator=NOT  AllPortsSameDT=off  OutDataTypeStr=boolean
  Logical Operator5 : Logic  Inputs=3  AllPortsSameDT=off  OutDataTypeStr=boolean
  Logical Operator6 : Logic  Operator=NOT  AllPortsSameDT=off  OutDataTypeStr=boolean
  Logical Operator8 : Logic  Operator=OR  AllPortsSameDT=off  OutDataTypeStr=boolean
  Relay : Relay  OnSwitchValue=ONE_INT  OffSwitchValue=ZERO_INT
  SR_Latch1 : Subsystem  mask(SR_Latch){}
      mask help: SR latch function.
  SR_Latch3 : hcu_lib/Basic_Blocks/SR_Latch
  SR_Latch4 : hcu_lib/Basic_Blocks/SR_Latch
  Switch{,1,4..7} (6 alike) : Switch  Criteria=u2 ~= 0
  Switch3 : Switch  Commented=on  Criteria=u2 ~= 0
  Test Detection Criteria : hcu_lib/Basic_Blocks/Test Detection Criteria
  Timer1 : hcu_lib/Basic_Blocks/Timer
  Unit Delay3 : UnitDelay  Commented=on  SampleTime=-1  HasFrameUpgradeWarning=on
  VDDM_C3BMS6CSDTC_raw32 : Outport
  VDDM_C3BMS6CSCFS_flg : Outport  Port=2
  wires:
  No_CAN3_BUS_OFF/1 -> [No_CAN3_BUS_OFF]
  VPMM_PowerSta_enum/1 -> [VPMM_PowerSta_enum]
  VPMM_PwrStaSW_enum/1 -> [VPMM_PwrStaSW_enum]
  VDDM_C3BMS6CSChk_flg/1 -> [VDDM_C3BMS6CSChk_flg]
  task_time_s/1 -> [task_time_s]
  Demux/1 -> Unit Delay3/1
  Logical Operator15/1 -> DTC_Couter/2
  Logical Operator18/1 -> [VDDM_C3BMS6CSCFS_flg]
  SR_Latch4/1 -> Logical Operator18/1
  DTC_Couter/1 -> SR_Latch4/1
  Constant46/1 -> Logical Operator19/2
  [VDDM_C3BMS6CSCFSRls_flg] -> Logical Operator3/2
  [VDDM_C3BMS6CSPass_flg] -> Logical Operator3/1
  Switch3/1 -> Demux/1
  Data Type Conversion1/1 -> [VDDM_C3BMS6CSDTC_cnt]  "VDDM_C3BMS6CSDTC_cnt"
  Equal3/1 -> SR_Latch1/1(set)
  SR_Latch3/1 -> Logical Operator12/2
  Logical Operator3/1 -> Logical Operator15/1
  [VDDM_C3BMS6CSDFSRls_flg] -> Logical Operator21/1
  Constant18/1 -> Timer1/4
  Constant15/1 -> Logical Operator18/2
  Constant22/1 -> Switch7/1
  Constant4/1 -> Equal4/2
  Timer1/1 -> Equal3/1
  [VDDM_C3BMS6CSDet_flg] -> Logical Operator19/1
  [VDDM_C3BMS6CSCFSRls_flg] -> SR_Latch4/2
  Switch/1 -> Goto16/1
  Relay/1 -> SR_Latch3/1
  Logical Operator6/1 -> Timer1/1
  Constant24/1 -> Switch4/1
  [VDDM_C3BMS6CSPass_flg] -> Switch7/2
  DTC_Couter/2 -> Data Type Conversion1/1
  Constant48/1 -> DTC_Couter/3
  Equal4/1 -> Logical Operator8/1
  Logical Operator19/1 -> DTC_Couter/1
  Constant20/1 -> Logical Operator12/1
  Switch4/1 -> [VDDM_C3BMS6CSCFSRls_flg]
  SR_Latch1/1(latched) -> [VDDM_C3BMS6CSPass_flg]
  Logical Operator12/1 -> [VDDM_C3BMS6CSDFS_flg]
  [No_CAN3_BUS_OFF] -> Logical Operator2/1
  Constant16/1 -> Switch6/3
  Constant28/1 -> Switch5/3
  [VDDM_C3BMS6CSDTC_cnt] -> Relay/1
  Logical Operator21/1 -> SR_Latch3/2
  Logical Operator8/1 -> Switch4/2
  From13/1 -> Switch3/2
  [DTC_clear_request] -> Logical Operator8/2
  Constant23/1 -> Switch7/3
  [VDDM_C3BMS6CSCFS_flg] -> Logical Operator21/2
  Constant25/1 -> Switch4/3
  [VDDM_C3BMS6CSChk_flg] -> Switch6/1
  Constant5/1 -> Logical Operator15/2
  [VDDM_xxx_flg] -> SR_Latch1/2(reset)
  Switch7/1 -> [VDDM_C3BMS6CSDFSRls_flg]
  Constant21/1 -> Switch/3
  Equal/1 -> Logical Operator2/2
  Logical Operator2/1 -> Switch5/2
  Constant19/1 -> Equal3/2
  Constant26/1 -> Equal/2
  [VDDM_C3BMS6CSChk_flg] -> Switch5/1
  [task_time_s] -> Test Detection Criteria/2
  Constant40/1 -> Test Detection Criteria/3
  Test Detection Criteria/1 -> [VDDM_C3BMS6CSDet_flg]  "VDDM_C3BMS6CSDet_flg"
  Switch6/1 -> Logical Operator6/1, Timer1/2
  Constant3/1 -> Switch/1
  [VDDM_C3BMS6CSCFS_flg] -> Switch/2
  DTC_clear_request/1 -> [DTC_clear_request]
  VDDM_C3BMS6LCCFS_flg/1 -> [VDDM_C3BMS6LCCFS_flg]
  [VDDM_C3BMS6LCCFS_flg] -> Logical Operator1/1
  Logical Operator1/1 -> Logical Operator2/3
  Constant1/1 -> Equal1/2
  Equal1/1 -> Logical Operator5/2
  [No_CAN3_BUS_OFF] -> Logical Operator5/1
  Logical Operator5/1 -> Switch6/2
  [VDDM_C3BMS6LCCFS_flg] -> Logical Operator4/1
  Logical Operator4/1 -> Logical Operator5/3
  [VPMM_PowerSta_enum] -> Equal4/1
  [VPMM_PwrStaSW_enum] -> Equal/1
  [VPMM_PwrStaSW_enum] -> Equal1/1
  [task_time_s] -> Timer1/3
  [VDDM_C3BMS6CSPass_flg] -> DTC_Info/2
  [VDDM_C3BMS6CSCFS_flg] -> DTC_Info/3
  DTC_Info/1 -> VDDM_C3BMS6CSDTC_raw32/1  "VDDM_C3BMS6CSDTC_raw32"
  [VDDM_C3BMS6CSDet_flg] -> DTC_Info/1
  Constant41/1 -> Test Detection Criteria/4
  [DTC_clear_request] -> DTC_Info/4
  [DTC_clear_request] -> Switch1/2
  Switch1/1 -> Test Detection Criteria/1
  Switch5/1 -> [VDDM_xxx_flg], Switch1/3
  Constant2/1 -> Switch1/1
  [VDDM_C3BMS6CSCFS_flg] -> VDDM_C3BMS6CSCFS_flg/1
